simulink model "pv_Bypass_characteristic"  (R2024b)
settings: Solver=ode5  StartTime=0.0  StopTime=5  RelTol=1e-3
libraries: spsPVArrayLib x4, spsDiodeLib x3, spsCurrentMeasurementLib x2, simulink x2, spsVoltageMeasurementLib x2, spsControlledCurrentSourceLib x1, spsControlledVoltageSourceLib x1, spspowerguiLib x1
settings Model: Creator=30698  LastModifiedBy=strat
settings RTWCC: GPUComputeCapability=3.5

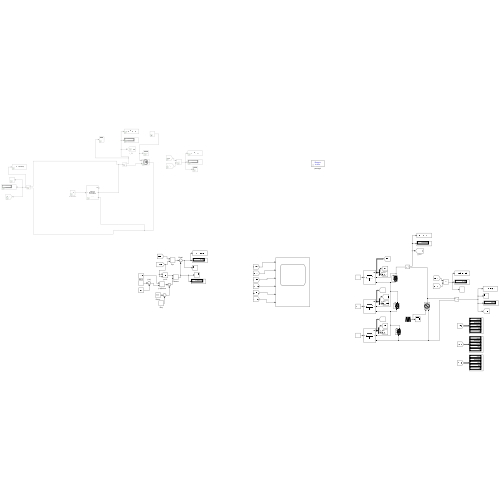
[thumbnail: Simulink's stored preview of the top-level diagram]
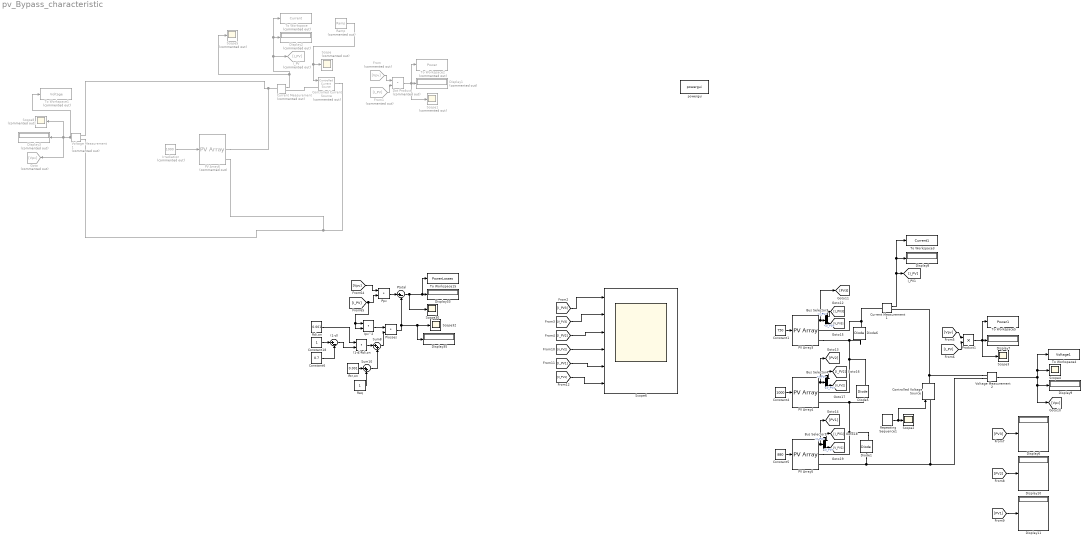
== system pv_Bypass_characteristic ==
  (1-d) : Sum  Inputs=|+-
  (1-d)Rdi,on : DotProduct  OutDataTypeStr=Inherit: Inherit via internal rule
  Bus Selector3 : BusSelector  OutputSignals=I_PV,V_PV
  Bus Selector4 : BusSelector  OutputSignals=I_PV,V_PV
  Bus Selector5 : BusSelector  OutputSignals=I_PV,V_PV
  Constant1 : Constant  Value=750
  Constant18 : Constant
  Constant4 : Constant  Value=1000
  Constant5 : Constant  Value=880
  Constant6 : Constant  Value=0.7
  Controlled Current Source : spsControlledCurrentSourceLib/Controlled Current Source  Commented=on  Initialize=off  Source_Type=AC  Amplitude=0  Phase=0  Frequency=0  Measurements=None
  Controlled Voltage Source : spsControlledVoltageSourceLib/Controlled Voltage Source  Initialize=on  Source_Type=AC  Amplitude=0  Phase=0  Frequency=0  Measurements=None
  Current Measurement : spsCurrentMeasurementLib/Current Measurement  Commented=on  PhasorSimulation=off  OutputType=Complex  PSBequivalent=0
  Current Measurement1 : spsCurrentMeasurementLib/Current Measurement  PhasorSimulation=off  OutputType=Complex  PSBequivalent=0
  Diode1 : spsDiodeLib/Diode  Ron=0.001  Lon=0  Vf=0.8  IC=0  UseSnubber=0  Rs=500  Cs=250e-9  Measurements=on
  Diode5 : spsDiodeLib/Diode  Ron=0.001  Lon=0  Vf=0.8  IC=0  UseSnubber=0  Rs=500  Cs=250e-9  Measurements=on
  Diode6 : spsDiodeLib/Diode  Ron=0.001  Lon=0  Vf=0.8  IC=0  UseSnubber=0  Rs=500  Cs=250e-9  Measurements=on
  Display1 : Display  Commented=on
  Display{6..11,33,35} (8 alike) : Display
  Display2 : Display  Commented=on
  Display3 : Display  Commented=on
  Dot Product : DotProduct  Commented=on  OutDataTypeStr=Inherit: Inherit via internal rule
  From : From  Commented=on  GotoTag=Vpv
  From1 : From  Commented=on  GotoTag=I_PV
  Goto : Goto  Commented=on  GotoTag=Vpv
  I_PV : Goto  Commented=on  GotoTag=I_PV
  Ipv^2 : DotProduct  OutDataTypeStr=Inherit: Inherit via internal rule
  Irradiation : Constant  Commented=on  Value=1000
  PV Array3 : spsPVArrayLib/PV Array  Npar=10  Nser=5  PlotType=array @ 1000 W/m2 & specified temperatures  S_vec="[ 1000  500  100 ]"  Temp_C_vec="[ 45 25  ]"  ModuleName=User-defined  PlotWhenSelected=off  Pm=213.15  Ncell=60  Voc=36.3  Isc=7.84  Vm=29  Im=7.35  beta_Voc_pc=-0.36099  alpha_Isc_pc=0.102  beta_Voc=-0.13104  alpha_Isc=0.0079968  IL=7.8654  I0=2.9273e-10  nI=0.98119  Rsh=313.0553  Rs=0.39381  RobustModel=on  RobustCellTemperature=25  BAL=on  Tc=1e-6  Tfilter=5e-5
  PV Array4 : spsPVArrayLib/PV Array  Npar=10  Nser=5  PlotType=array @ 1000 W/m2 & specified temperatures  S_vec="[ 1000  500  100 ]"  Temp_C_vec="[ 45 25  ]"  ModuleName=User-defined  PlotWhenSelected=off  Pm=213.15  Ncell=60  Voc=36.3  Isc=7.84  Vm=29  Im=7.35  beta_Voc_pc=-0.36099  alpha_Isc_pc=0.102  beta_Voc=-0.13104  alpha_Isc=0.0079968  IL=7.8654  I0=2.9273e-10  nI=0.98119  Rsh=313.0553  Rs=0.39381  RobustModel=on  RobustCellTemperature=25  BAL=on  Tc=1e-6  Tfilter=5e-5
  PV Array5 : spsPVArrayLib/PV Array  Npar=10  Nser=5  PlotType=array @ 1000 W/m2 & specified temperatures  S_vec="[ 1000  500  100 ]"  Temp_C_vec="[ 45 25  ]"  ModuleName=User-defined  PlotWhenSelected=off  Pm=213.15  Ncell=60  Voc=36.3  Isc=7.84  Vm=29  Im=7.35  beta_Voc_pc=-0.36099  alpha_Isc_pc=0.102  beta_Voc=-0.13104  alpha_Isc=0.0079968  IL=7.8654  I0=2.9273e-10  nI=0.98119  Rsh=313.0553  Rs=0.39381  RobustModel=on  RobustCellTemperature=25  BAL=on  Tc=1e-6  Tfilter=5e-5
  PV Array6 : spsPVArrayLib/PV Array  Commented=on  Npar=5  Nser=20.68  PlotType=array @ 25 deg.C & specified irradiances  S_vec="[ 1000  900  800 ]"  Temp_C_vec="[ 45 25  ]"  ModuleName=User-defined  PlotWhenSelected=off  Pm=217.5  Ncell=60  Voc=34.7  Isc=7.84  Vm=29  Im=7.5  beta_Voc_pc=-0.36099  alpha_Isc_pc=0.102  beta_Voc=-0.12526  alpha_Isc=0.0079968  IL=7.8839  I0=2.9416e-10  nI=0.93761  Rsh=1134.9167  Rs=0.18184  RobustModel=on  RobustCellTemperature=25  BAL=on  Tc=1e-6  Tfilter=5e-5
  Plosses : DotProduct  OutDataTypeStr=Inherit: Inherit via internal rule
  Ppv : DotProduct  OutDataTypeStr=Inherit: Inherit via internal rule
  Product1 : Product
  Ptotal : Sum  Inputs=|+-
  Ramp : simulink/Sources/Ramp  Commented=on  slope=39.413  start=0  InitialOutput=0
  Rdi,on : Constant  Value=0.001
  Repeating Sequence1 : simulink/Sources/Repeating Sequence  rep_seq_t=[0 1 2]  rep_seq_y=[0 541.349 0]
  Req : Constant
  Rtr,on : Constant  Value=0.001
  Scope{,1,5,8} (4 alike) : Scope  Commented=on
  Scope{2..4,30,32} (5 alike) : Scope
  Scope6 : Scope  NumInputPorts=6
  Sum10 : Sum  Inputs=|++
  Sum8 : Sum  Inputs=|++
  To Workspace : ToWorkspace  Commented=on  VariableName=Current  SampleTime=-1
      settings: Save2DSignal=2-D array (concatenate along first dimension)
  To Workspace1 : ToWorkspace  Commented=on  VariableName=Voltage  SampleTime=-1
      settings: Save2DSignal=2-D array (concatenate along first dimension)
  To Workspace15 : ToWorkspace  VariableName=PowerLosses  SampleTime=-1
      settings: Save2DSignal=2-D array (concatenate along first dimension)
  To Workspace2 : ToWorkspace  Commented=on  VariableName=Power  SampleTime=-1
      settings: Save2DSignal=2-D array (concatenate along first dimension)
  To Workspace3 : ToWorkspace  VariableName=Current1  SampleTime=-1
      settings: Save2DSignal=2-D array (concatenate along first dimension)
  To Workspace4 : ToWorkspace  VariableName=Voltage1  SampleTime=-1
      settings: Save2DSignal=2-D array (concatenate along first dimension)
  To Workspace5 : ToWorkspace  VariableName=Power1  SampleTime=-1
      settings: Save2DSignal=2-D array (concatenate along first dimension)
  Voltage Measurement1 : spsVoltageMeasurementLib/Voltage Measurement  Commented=on  PhasorSimulation=off  OutputType=Complex  PSBequivalent=0
  Voltage Measurement2 : spsVoltageMeasurementLib/Voltage Measurement  PhasorSimulation=off  OutputType=Complex  PSBequivalent=0
  powergui : spspowerguiLib/powergui  Priority=1  SimulationMode=Discrete  SampleTime=1e-5  frequency=60  Iterations=50  frequencyindice=0  Pbase=100e6  ErrMax=1e-4  UnitsV=kV  UnitsW=MW  buscounter=0  FunctionMessages=off  echomessages=off  EnableUseOfTLC=off  CurrentSourceSwitches=off  DisableSnubberDevices=off  DisableRonSwitches=off  DisableVfSwitches=off  DisplayEquations=off  AutomaticDiscreteSolvers=off  SolverType=Tustin/Backward Euler (TBE)  Interpol=off  ExternalGateDelay=off  methode=off  Ts=100  x0status=blocks  SPID=on  SwTol=0  HookPort=off  NonlinearTolerance=1e-4  nMaxIteration=100  ContinueOnMaxIteration=off  RestoreLinks=warning  ResistiveCurrentMeasurement=off  Frange=[0:2:500]  Ylog=off  Xlog=on  ShowGrid=off  save=off  variable=ZData  structure=0  ZoomFFT=off  StartTime=0.0  cycles=1  DisplayStyle=1  fundamental=60  FreqAxis=off  MaxFrequency=1000  frequencyindicesteady=1  RmsSteady=1  display=off
  wires:
  Current Measurement/1 -> Scope5/1, To Workspace/1, Display2/1, I_PV/1
  Voltage Measurement1/1 -> To Workspace1/1, Scope8/1, Display3/1, Goto/1
  From/1 -> Dot Product/1
  From1/1 -> Dot Product/2
  Dot Product/1 -> To Workspace2/1, Scope1/1, Display1/1
  Product1/1 -> Scope3/1, Display7/1, To Workspace5/1
  PV Array3/1 -> [PV3], Bus Selector3/1
  [PV2] -> Display10/1
  [PV1] -> Display11/1
  Constant1/1 -> PV Array3/1
  PV Array4/1 -> [PV2], Bus Selector4/1
  Bus Selector5/1 -> [I_PV1]  "<I_PV>"
  Bus Selector5/2 -> [V_PV1]  "<V_PV>"
  [PV3] -> Display6/1
  [Vpv] -> Product1/1
  Constant4/1 -> PV Array4/1
  Bus Selector3/2 -> [V_PV3]  "<V_PV>"
  Bus Selector4/1 -> [I_PV2]  "<I_PV>"
  PV Array5/1 -> [PV1], Bus Selector5/1
  [I_PV] -> Product1/2
  Bus Selector3/1 -> [I_PV3]  "<I_PV>"
  Voltage Measurement2/1 -> Display9/1, [Vpv], Scope4/1, To Workspace4/1
  Constant5/1 -> PV Array5/1
  Current Measurement1/1 -> [I_PV], Display8/1, To Workspace3/1
  Bus Selector4/2 -> [V_PV2]  "<V_PV>"
  Repeating Sequence1/1 -> Controlled Voltage Source/1, Scope2/1
  Ramp/1 -> Controlled Current Source/1, Scope/1
  Sum10/1 -> Sum8/2
  Ipv^2/1 -> Plosses/1
  Req/1 -> Sum10/2
  Rtr,on/1 -> Sum10/1
  (1-d)/1 -> (1-d)Rdi,on/2
  Ppv/1 -> Ptotal/1
  Constant6/1 -> (1-d)/2
  Rdi,on/1 -> (1-d)Rdi,on/1
  (1-d)Rdi,on/1 -> Sum8/1
  Constant18/1 -> (1-d)/1
  Sum8/1 -> Plosses/2
  [I_PV] -> Ipv^2/2, Ipv^2/1, Ppv/2
  Plosses/1 -> Ptotal/2, Display35/1, Scope32/1
  [Vpv] -> Ppv/1
  Ptotal/1 -> To Workspace15/1, Display33/1, Scope30/1
  Irradiation/1 -> PV Array6/1
  [I_PV3] -> Scope6/1
  [V_PV3] -> Scope6/2
  [I_PV2] -> Scope6/3
  [V_PV2] -> Scope6/4
  [I_PV1] -> Scope6/5
  [V_PV1] -> Scope6/6
  connections:
  Controlled Current Source/RConn1 -- Voltage Measurement1/LConn2 -- PV Array6/RConn2
  Controlled Current Source/LConn1 -- Current Measurement/RConn1
  Voltage Measurement2/LConn2 -- PV Array5/RConn2 -- Diode1/LConn1 -- Controlled Voltage Source/LConn1
  Diode1/RConn1 -- PV Array4/RConn2 -- Diode5/LConn1 -- PV Array5/RConn1
  PV Array4/RConn1 -- Diode5/RConn1 -- Diode6/LConn1 -- PV Array3/RConn2
  Voltage Measurement2/LConn1 -- Current Measurement1/RConn1 -- Controlled Voltage Source/RConn1
  PV Array3/RConn1 -- Current Measurement1/LConn1 -- Diode6/RConn1
  Voltage Measurement1/LConn1 -- PV Array6/RConn1 -- Current Measurement/LConn1
